simulink model "fuzzy_adaptive_sliding_mode"  (R2019b)
settings: Solver=VariableStepAuto  StartTime=0.0  StopTime=10.0  RelTol=1e-3
settings Model: Creator=Alien  LastModifiedBy=Alien

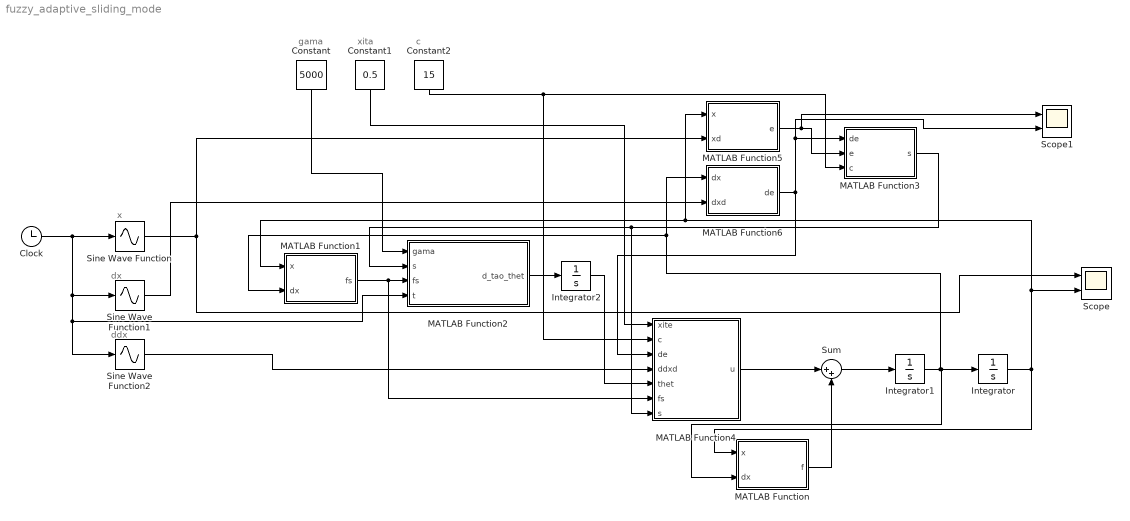
== system fuzzy_adaptive_sliding_mode ==
  note: c
  note: xita
  note: gama
  note: ddx
  note: x
  note: dx
  Clock : Clock
  Constant : Constant  Value=5000
  Constant1 : Constant  Value=0.5
  Constant2 : Constant  Value=15
  Integrator : Integrator
  Integrator1 : Integrator  InitialCondition=0.15
  Integrator2 : Integrator
  MATLAB Function : MATLAB Function  TreatAsAtomicUnit=on
  MATLAB Function1 : MATLAB Function  TreatAsAtomicUnit=on
  MATLAB Function2 : MATLAB Function  TreatAsAtomicUnit=on
  MATLAB Function3 : MATLAB Function  TreatAsAtomicUnit=on
  MATLAB Function4 : MATLAB Function  TreatAsAtomicUnit=on
  MATLAB Function5 : MATLAB Function  TreatAsAtomicUnit=on
  MATLAB Function6 : MATLAB Function  TreatAsAtomicUnit=on
  Scope : Scope  NumInputPorts=2
  Scope1 : Scope  NumInputPorts=2
  Sine Wave Function : Sin  TimeSource=Use external signal  SampleTime=0
  Sine Wave Function1 : Sin  TimeSource=Use external signal  Phase=pi/2  SampleTime=0
  Sine Wave Function2 : Sin  TimeSource=Use external signal  Amplitude=-1  SampleTime=0
  Sum : Sum  Inputs=|++
  wires:
  Integrator1/1 -> MATLAB Function1/2(dx), MATLAB Function6/1(dx), MATLAB Function/2(dx), Integrator/1
  Sum/1 -> Integrator1/1
  MATLAB Function/1(f) -> Sum/2
  MATLAB Function4/1(u) -> Sum/1
  MATLAB Function5/1(e) -> Scope1/1, MATLAB Function3/2(e)
  MATLAB Function6/1(de) -> MATLAB Function4/3(de), Scope1/2, MATLAB Function3/1(de)
  MATLAB Function3/1(s) -> MATLAB Function4/7(s), MATLAB Function2/2(s)
  Integrator/1 -> Scope/2, MATLAB Function1/1(x), MATLAB Function5/1(x), MATLAB Function/1(x)
  Clock/1 -> Sine Wave Function2/1, MATLAB Function2/4(t), Sine Wave Function1/1, Sine Wave Function/1
  MATLAB Function1/1(fs) -> MATLAB Function2/3(fs), MATLAB Function4/6(fs)
  Constant/1 -> MATLAB Function2/1(gama)
  Sine Wave Function2/1 -> MATLAB Function4/4(ddxd)
  Constant2/1 -> MATLAB Function3/3(c), MATLAB Function4/2(c)
  Constant1/1 -> MATLAB Function4/1(xite)
  Sine Wave Function/1 -> Scope/1, MATLAB Function5/2(xd)
  Sine Wave Function1/1 -> MATLAB Function6/2(dxd)
  MATLAB Function2/1(d_tao_thet) -> Integrator2/1
  Integrator2/1 -> MATLAB Function4/5(thet)

== matlab function fuzzy_adaptive_sliding_mode/MATLAB Function1 ==
  data: x input; fs output size=[25 1]; dx input
function fs = fcn(x, dx)
fs1 = 0; fs2 = ones(25,1);
u1 = ones(5,1); u2 = ones(5,1);
for l1 = 1:1:5
    u1(l1,1) = exp(-((x + pi/3 - (l1 - 1) * pi/6)/(pi/12))^2);
    u2(l1,1) = exp(-((dx + pi/3 - (l1 - 1) * pi/6)/(pi/12))^2);
end

for l1 = 1:1:5
    for l2 = 1:1:5
        fs2(5*(l1-1)+l2,1) = u1(l1,1) * u2(l2,1); %25*1
        fs1 = fs1 + u1(l1,1) * u2(l2,1);
    end
end

fs = fs2/(fs1+0.001);

== matlab function fuzzy_adaptive_sliding_mode/MATLAB Function ==
  data: x input; f output; dx input
function f = fcn(x, dx)
f = 10 * x * dx;

== matlab function fuzzy_adaptive_sliding_mode/MATLAB Function2 ==
  data: gama input; d_tao_thet output size=[25 1]; s input; fs input; t input
function d_tao_thet = fcn(gama, s, fs, t)
if t == 0
    d_tao_thet = ones(25,1)/10;
else
    d_tao_thet = gama * s * fs; %25*1
end

== matlab function fuzzy_adaptive_sliding_mode/MATLAB Function3 ==
  data: de input; s output; e input; c input
function s = fcn(de, e, c)
s = de + c*e;

== matlab function fuzzy_adaptive_sliding_mode/MATLAB Function4 ==
  data: xite input; u output; c input; de input; ddxd input; thet input; fs input; s input
function u = fcn(xite, c, de, ddxd, thet, fs, s)
fxp = thet' * fs;
u = -c * de + ddxd - fxp - xite * sign(s);

== matlab function fuzzy_adaptive_sliding_mode/MATLAB Function5 ==
  data: x input; e output; xd input
function e = fcn(x, xd)
e = x - xd;

== matlab function fuzzy_adaptive_sliding_mode/MATLAB Function6 ==
  data: dx input; de output; dxd input
function de = fcn(dx, dxd)
de = dx - dxd;
